simulink model "FDIA_Toolbox"  (R2018a)
settings: Solver=VariableStepAuto  StartTime=0.0  StopTime=10.0  RelTol=1e-3
libraries: commrandsrc3 x30, commutil2 x12, simulink_extras x6, simulink x4, commsynccomp2 x2, commanapbnd3 x2
(part 2 of 2)

== system FDIA_Toolbox/  /Attack Injected System2/valve ==
  control : Inport
  source flow : Inport  Port=2
  Limited Integrator : Subsystem  mask(Limited integrator.){lb=0, ub=1, xi=InitialPosition}
      mask prompts: lb "Lower bound:"; ub "Upper bound:"; xi "Initial condition"
      mask help: Limited integrator
      mask Help: Implements a limited integrator with \nan expression of the form:\n\nif(x<=lb and u<0) or (x>=ub and u>0)\n\txdot=0\nelse\n\txdot=u.
      mask Display: plot(-1,-0.2,3.5,1.2,[0.05,1,2,2.9],[0,0,1,1]);disp(' 1/s    ')
  Product : Product  SaturateOnIntegerOverflow=on  RndMeth=Zero  InputSameDT=on  OutDataTypeStr=Inherit: Same as first input
  out flow : Outport  InitialOutput=0
  wires:
  source flow/1 -> Product/2
  Product/1 -> out flow/1
  control/1 -> Limited Integrator/1(In_1)
  Limited Integrator/1(Out_1) -> Product/1

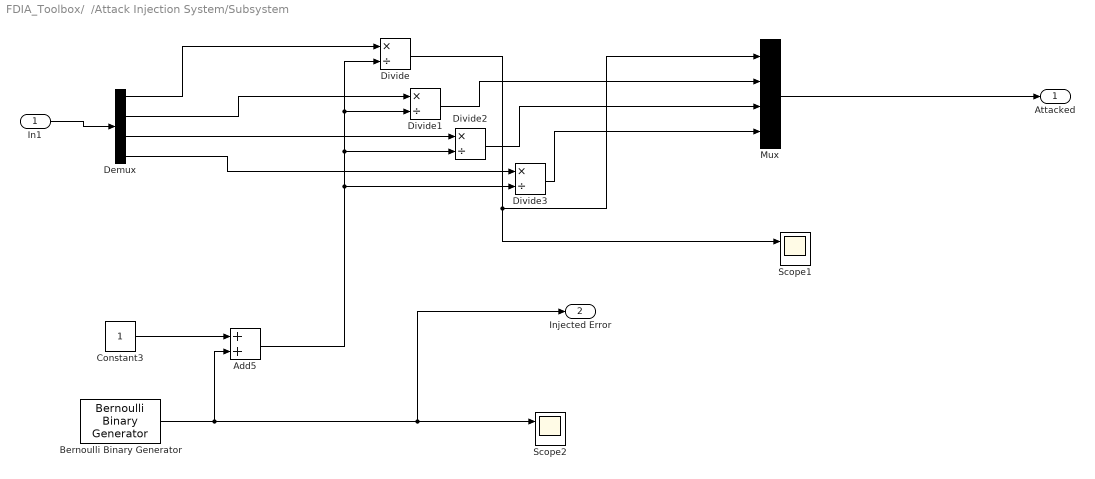
== system FDIA_Toolbox/  /Attack Injection System/Subsystem ==
  In1 : Inport
  Add5 : Sum  AccumDataTypeStr=uint8  RndMeth=Round
  Bernoulli Binary Generator : commrandsrc3/Bernoulli Binary Generator  ProbabilityOfZero=0.9  SeedSource=Auto  Seed=0  SampleTime=1  SamplesPerFrame=1  OutputDataType=uint8  SimulateUsing=Interpreted execution
  Constant3 : Constant  OutDataTypeStr=uint8
  Demux : Demux
  Divide{,1..3} (4 alike) : Product  Inputs=*/
  Mux : Mux
  Scope1 : Scope  NumInputPorts=2
  Scope2 : Scope  NumInputPorts=2
  Attacked : Outport
  Injected Error : Outport  Port=2
  wires:
  Demux/3 -> Divide2/1
  Demux/2 -> Divide1/1
  Demux/4 -> Divide3/1
  In1/1 -> Demux/1
  Mux/1 -> Attacked/1
  Divide/1 -> Scope1/1, Mux/1
  Bernoulli Binary Generator/1 -> Add5/2, Injected Error/1, Scope2/1
  Constant3/1 -> Add5/1
  Demux/1 -> Divide/1
  Add5/1 -> Divide3/2, Divide2/2, Divide1/2, Divide/2
  Divide1/1 -> Mux/2
  Divide2/1 -> Mux/3
  Divide3/1 -> Mux/4

== system FDIA_Toolbox/  /Attack Injection System1/tank  ==
  flow in : Inport
  1/area : Gain  Gain=1/area  SaturateOnIntegerOverflow=on  OutDataTypeStr=Inherit: Same as input  ParamDataTypeStr=Inherit: Same as input
  Overflow sensor1 : Relay  OnSwitchValue=ht - overflowLimit  OffSwitchValue=ht - overflowLimit  OnOutputValue=3  ZeroCross=off
  outletArea : Gain  Gain=outletArea  SaturateOnIntegerOverflow=on  OutDataTypeStr=Inherit: Same as input  ParamDataTypeStr=Inherit: Same as input
  sqrt(2gh) : Fcn  Expr=sqrt(2*9.8*u)
  sum : Sum  Inputs=+-  SaturateOnIntegerOverflow=on  InputSameDT=on  OutDataTypeStr=Inherit: Same as first input
  tank volume : Subsystem  mask(Limited integrator.){lb=0, ub=ht * area, xi=initialHt * area}
      mask prompts: lb "Lower bound:"; ub "Upper bound:"; xi "Initial condition"
      mask help: Limited integrator
      mask Help: Implements a limited integrator with \nan expression of the form:\n\nif(x<=lb and u<0) or (x>=ub and u>0)\n\txdot=0\nelse\n\txdot=u.
      mask Display: plot(-1,-0.2,3.5,1.2,[0.05,1,2,2.9],[0,0,1,1]);disp(' 1/s    ')
  water level : Outport  InitialOutput=0
  flow out : Outport  Port=2  InitialOutput=0
  overflow flag1 : Outport  Port=3  InitialOutput=0
  wires:
  outletArea/1 -> sum/2, flow out/1
  sqrt(2gh)/1 -> outletArea/1
  tank volume/1(Out_1) -> 1/area/1
  flow in/1 -> sum/1
  sum/1 -> tank volume/1(In_1)
  Overflow sensor1/1 -> overflow flag1/1
  1/area/1 -> sqrt(2gh)/1, Overflow sensor1/1, water level/1

== system FDIA_Toolbox/  /Attack Injection System1/valve ==
  control : Inport
  source flow : Inport  Port=2
  Limited Integrator : Subsystem  mask(Limited integrator.){lb=0, ub=1, xi=InitialPosition}
      mask prompts: lb "Lower bound:"; ub "Upper bound:"; xi "Initial condition"
      mask help: Limited integrator
      mask Help: Implements a limited integrator with \nan expression of the form:\n\nif(x<=lb and u<0) or (x>=ub and u>0)\n\txdot=0\nelse\n\txdot=u.
      mask Display: plot(-1,-0.2,3.5,1.2,[0.05,1,2,2.9],[0,0,1,1]);disp(' 1/s    ')
  Product : Product  SaturateOnIntegerOverflow=on  RndMeth=Zero  InputSameDT=on  OutDataTypeStr=Inherit: Same as first input
  out flow : Outport  InitialOutput=0
  wires:
  source flow/1 -> Product/2
  Product/1 -> out flow/1
  control/1 -> Limited Integrator/1(In_1)
  Limited Integrator/1(Out_1) -> Product/1

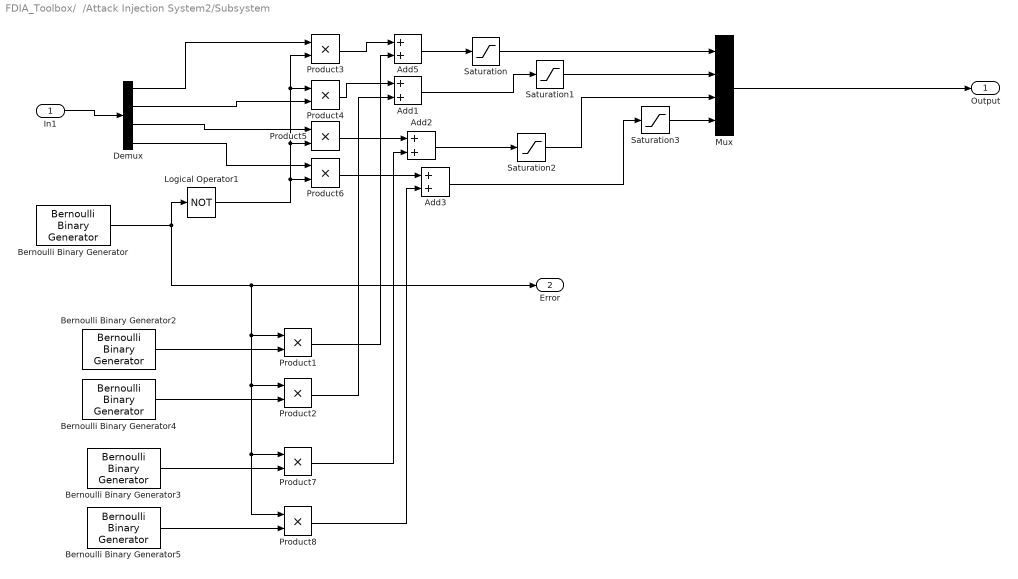
== system FDIA_Toolbox/  /Attack Injection System2/Subsystem ==
  In1 : Inport
  Add{1..3,5} (4 alike) : Sum  AccumDataTypeStr=uint8  RndMeth=Round
  Bernoulli Binary Generator : commrandsrc3/Bernoulli Binary Generator  ProbabilityOfZero=0.8  SeedSource=Auto  Seed=0  SampleTime=1  SamplesPerFrame=1  OutputDataType=uint8  SimulateUsing=Interpreted execution
  Bernoulli Binary Generator2 : commrandsrc3/Bernoulli Binary Generator  ProbabilityOfZero=0.1  SeedSource=Auto  Seed=0  SampleTime=1  SamplesPerFrame=1  OutputDataType=double  SimulateUsing=Interpreted execution
  Bernoulli Binary Generator3 : commrandsrc3/Bernoulli Binary Generator  ProbabilityOfZero=0.6  SeedSource=Auto  Seed=0  SampleTime=1  SamplesPerFrame=1  OutputDataType=double  SimulateUsing=Interpreted execution
  Bernoulli Binary Generator4 : commrandsrc3/Bernoulli Binary Generator  ProbabilityOfZero=0.4  SeedSource=Auto  Seed=0  SampleTime=1  SamplesPerFrame=1  OutputDataType=double  SimulateUsing=Interpreted execution
  Bernoulli Binary Generator5 : commrandsrc3/Bernoulli Binary Generator  ProbabilityOfZero=0.7  SeedSource=Auto  Seed=0  SampleTime=1  SamplesPerFrame=1  OutputDataType=double  SimulateUsing=Interpreted execution
  Demux : Demux
  Logical Operator1 : Logic  Operator=NOT  AllPortsSameDT=off  OutDataTypeStr=boolean
  Mux : Mux
  Product{1..8} (8 alike) : Product
  Saturation{,1..3} (4 alike) : Saturate  UpperLimit=1  LowerLimit=0
  Output : Outport
  Error : Outport  Port=2
  wires:
  Demux/3 -> Product5/1
  Demux/2 -> Product4/2
  Demux/4 -> Product6/1
  In1/1 -> Demux/1
  Mux/1 -> Output/1
  Bernoulli Binary Generator/1 -> Product8/1, Product7/1, Product2/1, Product1/1, Error/1, Logical Operator1/1
  Demux/1 -> Product3/1
  Logical Operator1/1 -> Product6/2, Product5/2, Product3/2, Product4/1
  Product3/1 -> Add5/1
  Product6/1 -> Add3/1
  Product5/1 -> Add2/1
  Product4/1 -> Add1/1
  Add5/1 -> Saturation/1
  Add1/1 -> Saturation1/1
  Add2/1 -> Saturation2/1
  Add3/1 -> Saturation3/1
  Saturation/1 -> Mux/1
  Saturation3/1 -> Mux/4
  Saturation2/1 -> Mux/3
  Saturation1/1 -> Mux/2
  Bernoulli Binary Generator5/1 -> Product8/2
  Product8/1 -> Add3/2
  Bernoulli Binary Generator3/1 -> Product7/2
  Product7/1 -> Add2/2
  Bernoulli Binary Generator4/1 -> Product2/2
  Product2/1 -> Add1/2
  Bernoulli Binary Generator2/1 -> Product1/2
  Product1/1 -> Add5/2

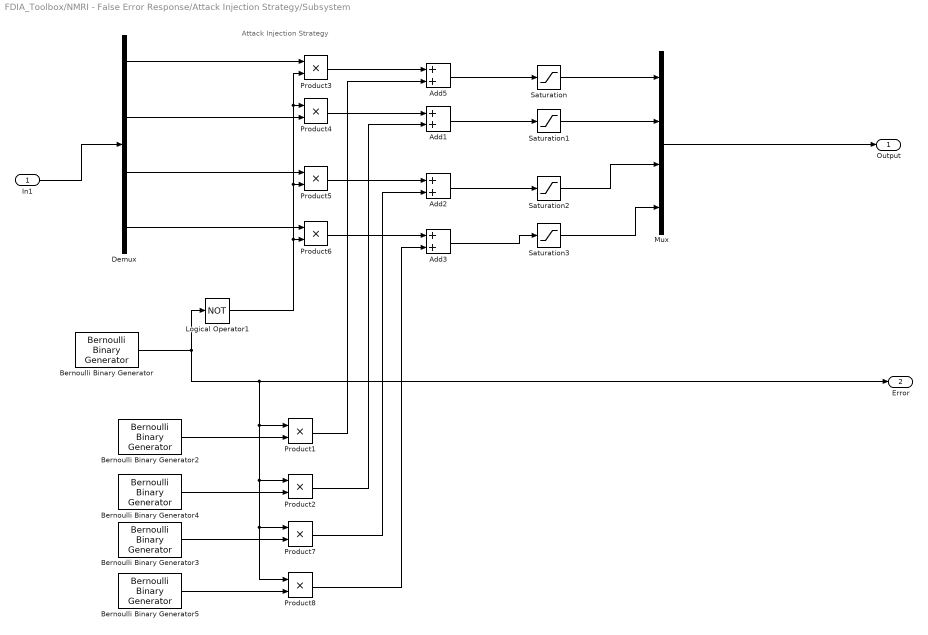
== system FDIA_Toolbox/NMRI - False Error Response/Attack Injection Strategy/Subsystem ==
  note: Attack Injection Strategy
  In1 : Inport
  Add{1..3,5} (4 alike) : Sum  AccumDataTypeStr=uint8  RndMeth=Round
  Bernoulli Binary Generator : commrandsrc3/Bernoulli Binary Generator  ProbabilityOfZero=0.8  SeedSource=Auto  Seed=0  SampleTime=1  SamplesPerFrame=1  OutputDataType=uint8  SimulateUsing=Interpreted execution
  Bernoulli Binary Generator2 : commrandsrc3/Bernoulli Binary Generator  ProbabilityOfZero=0.1  SeedSource=Auto  Seed=0  SampleTime=1  SamplesPerFrame=1  OutputDataType=double  SimulateUsing=Interpreted execution
  Bernoulli Binary Generator3 : commrandsrc3/Bernoulli Binary Generator  ProbabilityOfZero=0.6  SeedSource=Auto  Seed=0  SampleTime=1  SamplesPerFrame=1  OutputDataType=double  SimulateUsing=Interpreted execution
  Bernoulli Binary Generator4 : commrandsrc3/Bernoulli Binary Generator  ProbabilityOfZero=0.4  SeedSource=Auto  Seed=0  SampleTime=1  SamplesPerFrame=1  OutputDataType=double  SimulateUsing=Interpreted execution
  Bernoulli Binary Generator5 : commrandsrc3/Bernoulli Binary Generator  ProbabilityOfZero=0.7  SeedSource=Auto  Seed=0  SampleTime=1  SamplesPerFrame=1  OutputDataType=double  SimulateUsing=Interpreted execution
  Demux : Demux
  Logical Operator1 : Logic  Operator=NOT  AllPortsSameDT=off  OutDataTypeStr=boolean
  Mux : Mux
  Product{1..8} (8 alike) : Product
  Saturation{,1..3} (4 alike) : Saturate  UpperLimit=1  LowerLimit=0
  Output : Outport
  Error : Outport  Port=2
  wires:
  Demux/3 -> Product5/1
  Demux/2 -> Product4/2
  Demux/4 -> Product6/1
  In1/1 -> Demux/1
  Mux/1 -> Output/1
  Bernoulli Binary Generator/1 -> Logical Operator1/1, Product8/1, Product7/1, Product2/1, Product1/1, Error/1
  Demux/1 -> Product3/1
  Logical Operator1/1 -> Product6/2, Product5/2, Product3/2, Product4/1
  Product3/1 -> Add5/1
  Product6/1 -> Add3/1
  Product5/1 -> Add2/1
  Product4/1 -> Add1/1
  Add5/1 -> Saturation/1
  Add1/1 -> Saturation1/1
  Add2/1 -> Saturation2/1
  Add3/1 -> Saturation3/1
  Saturation/1 -> Mux/1
  Saturation3/1 -> Mux/4
  Saturation2/1 -> Mux/3
  Saturation1/1 -> Mux/2
  Bernoulli Binary Generator5/1 -> Product8/2
  Product8/1 -> Add3/2
  Bernoulli Binary Generator3/1 -> Product7/2
  Product7/1 -> Add2/2
  Bernoulli Binary Generator4/1 -> Product2/2
  Product2/1 -> Add1/2
  Bernoulli Binary Generator2/1 -> Product1/2
  Product1/1 -> Add5/2

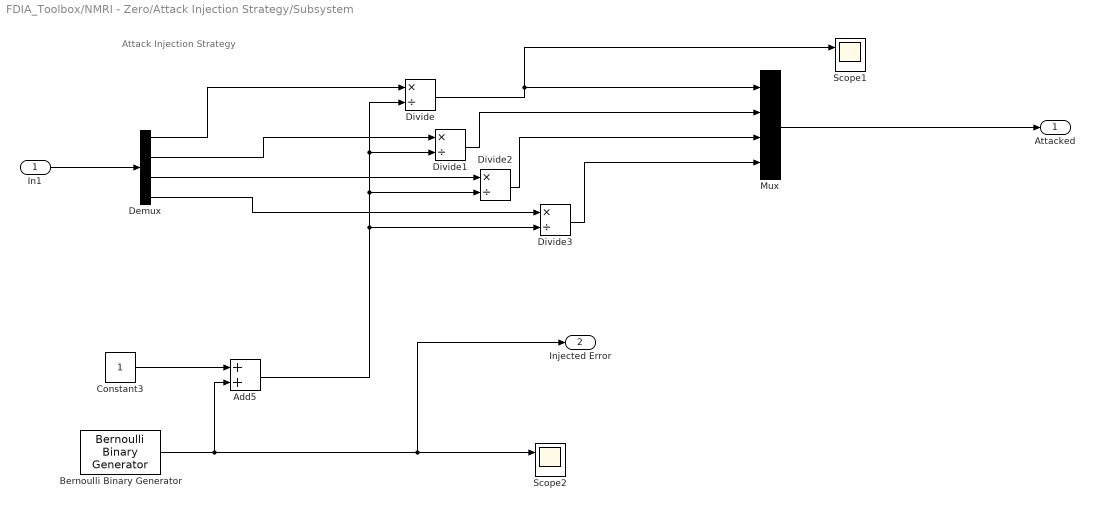
== system FDIA_Toolbox/NMRI - Zero/Attack Injection Strategy/Subsystem ==
  note: Attack Injection Strategy
  In1 : Inport
  Add5 : Sum  AccumDataTypeStr=uint8  RndMeth=Round
  Bernoulli Binary Generator : commrandsrc3/Bernoulli Binary Generator  ProbabilityOfZero=0.9  SeedSource=Auto  Seed=0  SampleTime=1  SamplesPerFrame=1  OutputDataType=uint8  SimulateUsing=Interpreted execution
  Constant3 : Constant  OutDataTypeStr=uint8
  Demux : Demux
  Divide{,1..3} (4 alike) : Product  Inputs=*/
  Mux : Mux
  Scope1 : Scope  NumInputPorts=2
  Scope2 : Scope  NumInputPorts=2
  Attacked : Outport
  Injected Error : Outport  Port=2
  wires:
  Demux/3 -> Divide2/1
  Demux/2 -> Divide1/1
  Demux/4 -> Divide3/1
  In1/1 -> Demux/1
  Mux/1 -> Attacked/1
  Divide/1 -> Mux/1, Scope1/1
  Bernoulli Binary Generator/1 -> Add5/2, Injected Error/1, Scope2/1
  Constant3/1 -> Add5/1
  Demux/1 -> Divide/1
  Add5/1 -> Divide3/2, Divide2/2, Divide1/2, Divide/2
  Divide1/1 -> Mux/2
  Divide2/1 -> Mux/3
  Divide3/1 -> Mux/4

== system FDIA_Toolbox/NMRI- Ones/Attack Induced Strategy/Subsystem ==
  note: Attack Injection Strategy
  In1 : Inport
  Demux : Demux
  Mux : Mux
  Saturation{,1..3} (4 alike) : Saturate  UpperLimit=1  LowerLimit=0
  Attacked Injection : Outport
  wires:
  Demux/3 -> Saturation2/1
  Demux/2 -> Saturation1/1
  In1/1 -> Demux/1
  Mux/1 -> Attacked Injection/1
  Demux/1 -> Saturation/1
  Demux/4 -> Saturation3/1
  Saturation/1 -> Mux/1
  Saturation3/1 -> Mux/4
  Saturation2/1 -> Mux/3
  Saturation1/1 -> Mux/2

== system FDIA_Toolbox/  /Attack Induced System1/tank /tank volume ==
  In_1 : Inport
  Fcn : Fcn  Expr=u[2]*((((u[1]>lb)+(u[2]>=0))>0) * (((u[1]<ub)+(u[2]<=0))>0))
  Integrator : Integrator  InitialCondition=xi
  Mux : Mux  Inputs=2
  Saturation : Saturate  UpperLimit=ub  LowerLimit=lb  ZeroCross=off
  Out_1 : Outport  InitialOutput=0
  wires:
  Integrator/1 -> Saturation/1, Mux/1
  Fcn/1 -> Integrator/1
  Mux/1 -> Fcn/1
  In_1/1 -> Mux/2
  Saturation/1 -> Out_1/1

== system FDIA_Toolbox/  /Attack Induced System1/valve/Limited Integrator ==
  In_1 : Inport
  Fcn : Fcn  Expr=u[2]*((((u[1]>lb)+(u[2]>=0))>0) * (((u[1]<ub)+(u[2]<=0))>0))
  Integrator : Integrator  InitialCondition=xi
  Mux : Mux  Inputs=2
  Saturation : Saturate  UpperLimit=ub  LowerLimit=lb  ZeroCross=off
  Out_1 : Outport  InitialOutput=0
  wires:
  Integrator/1 -> Saturation/1, Mux/1
  Fcn/1 -> Integrator/1
  Mux/1 -> Fcn/1
  In_1/1 -> Mux/2
  Saturation/1 -> Out_1/1

== system FDIA_Toolbox/  /Attack Injected System/tank /tank volume ==
  In_1 : Inport
  Fcn : Fcn  Expr=u[2]*((((u[1]>lb)+(u[2]>=0))>0) * (((u[1]<ub)+(u[2]<=0))>0))
  Integrator : Integrator  InitialCondition=xi
  Mux : Mux  Inputs=2
  Saturation : Saturate  UpperLimit=ub  LowerLimit=lb  ZeroCross=off
  Out_1 : Outport  InitialOutput=0
  wires:
  Integrator/1 -> Saturation/1, Mux/1
  Fcn/1 -> Integrator/1
  Mux/1 -> Fcn/1
  In_1/1 -> Mux/2
  Saturation/1 -> Out_1/1

== system FDIA_Toolbox/  /Attack Injected System/valve/Limited Integrator ==
  In_1 : Inport
  Fcn : Fcn  Expr=u[2]*((((u[1]>lb)+(u[2]>=0))>0) * (((u[1]<ub)+(u[2]<=0))>0))
  Integrator : Integrator  InitialCondition=xi
  Mux : Mux  Inputs=2
  Saturation : Saturate  UpperLimit=ub  LowerLimit=lb  ZeroCross=off
  Out_1 : Outport  InitialOutput=0
  wires:
  Integrator/1 -> Saturation/1, Mux/1
  Fcn/1 -> Integrator/1
  Mux/1 -> Fcn/1
  In_1/1 -> Mux/2
  Saturation/1 -> Out_1/1

== system FDIA_Toolbox/  /Attack Injected System2/Original System/tank 1 ==
  flow in : Inport
  1/area : Gain  Gain=1/area  SaturateOnIntegerOverflow=on  OutDataTypeStr=Inherit: Same as input  ParamDataTypeStr=Inherit: Same as input
  Overflow sensor1 : Relay  OnSwitchValue=ht - overflowLimit  OffSwitchValue=ht - overflowLimit  OnOutputValue=3  ZeroCross=off
  outletArea : Gain  Gain=outletArea  SaturateOnIntegerOverflow=on  OutDataTypeStr=Inherit: Same as input  ParamDataTypeStr=Inherit: Same as input
  sqrt(2gh) : Fcn  Expr=sqrt(2*9.8*u)
  sum : Sum  Inputs=+-  SaturateOnIntegerOverflow=on  InputSameDT=on  OutDataTypeStr=Inherit: Same as first input
  tank volume : Subsystem  mask(Limited integrator.){lb=0, ub=ht * area, xi=initialHt * area}
      mask prompts: lb "Lower bound:"; ub "Upper bound:"; xi "Initial condition"
      mask help: Limited integrator
      mask Help: Implements a limited integrator with \nan expression of the form:\n\nif(x<=lb and u<0) or (x>=ub and u>0)\n\txdot=0\nelse\n\txdot=u.
      mask Display: plot(-1,-0.2,3.5,1.2,[0.05,1,2,2.9],[0,0,1,1]);disp(' 1/s    ')
  water level : Outport  InitialOutput=0
  flow out : Outport  Port=2  InitialOutput=0
  overflow flag1 : Outport  Port=3  InitialOutput=0
  wires:
  outletArea/1 -> sum/2, flow out/1
  sqrt(2gh)/1 -> outletArea/1
  tank volume/1(Out_1) -> 1/area/1
  flow in/1 -> sum/1
  sum/1 -> tank volume/1(In_1)
  Overflow sensor1/1 -> overflow flag1/1
  1/area/1 -> sqrt(2gh)/1, Overflow sensor1/1, water level/1

== system FDIA_Toolbox/  /Attack Injected System2/Original System/valve1 ==
  control : Inport
  source flow : Inport  Port=2
  Limited Integrator : Subsystem  mask(Limited integrator.){lb=0, ub=1, xi=InitialPosition}
      mask prompts: lb "Lower bound:"; ub "Upper bound:"; xi "Initial condition"
      mask help: Limited integrator
      mask Help: Implements a limited integrator with \nan expression of the form:\n\nif(x<=lb and u<0) or (x>=ub and u>0)\n\txdot=0\nelse\n\txdot=u.
      mask Display: plot(-1,-0.2,3.5,1.2,[0.05,1,2,2.9],[0,0,1,1]);disp(' 1/s    ')
  Product : Product  SaturateOnIntegerOverflow=on  RndMeth=Zero  InputSameDT=on  OutDataTypeStr=Inherit: Same as first input
  out flow : Outport  InitialOutput=0
  wires:
  source flow/1 -> Product/2
  Product/1 -> out flow/1
  control/1 -> Limited Integrator/1(In_1)
  Limited Integrator/1(Out_1) -> Product/1

== system FDIA_Toolbox/  /Attack Injected System2/tank /tank volume ==
  In_1 : Inport
  Fcn : Fcn  Expr=u[2]*((((u[1]>lb)+(u[2]>=0))>0) * (((u[1]<ub)+(u[2]<=0))>0))
  Integrator : Integrator  InitialCondition=xi
  Mux : Mux  Inputs=2
  Saturation : Saturate  UpperLimit=ub  LowerLimit=lb  ZeroCross=off
  Out_1 : Outport  InitialOutput=0
  wires:
  Integrator/1 -> Saturation/1, Mux/1
  Fcn/1 -> Integrator/1
  Mux/1 -> Fcn/1
  In_1/1 -> Mux/2
  Saturation/1 -> Out_1/1

== system FDIA_Toolbox/  /Attack Injected System2/valve/Limited Integrator ==
  In_1 : Inport
  Fcn : Fcn  Expr=u[2]*((((u[1]>lb)+(u[2]>=0))>0) * (((u[1]<ub)+(u[2]<=0))>0))
  Integrator : Integrator  InitialCondition=xi
  Mux : Mux  Inputs=2
  Saturation : Saturate  UpperLimit=ub  LowerLimit=lb  ZeroCross=off
  Out_1 : Outport  InitialOutput=0
  wires:
  Integrator/1 -> Saturation/1, Mux/1
  Fcn/1 -> Integrator/1
  Mux/1 -> Fcn/1
  In_1/1 -> Mux/2
  Saturation/1 -> Out_1/1

== system FDIA_Toolbox/  /Attack Injection System1/tank /tank volume ==
  In_1 : Inport
  Fcn : Fcn  Expr=u[2]*((((u[1]>lb)+(u[2]>=0))>0) * (((u[1]<ub)+(u[2]<=0))>0))
  Integrator : Integrator  InitialCondition=xi
  Mux : Mux  Inputs=2
  Saturation : Saturate  UpperLimit=ub  LowerLimit=lb  ZeroCross=off
  Out_1 : Outport  InitialOutput=0
  wires:
  Integrator/1 -> Saturation/1, Mux/1
  Fcn/1 -> Integrator/1
  Mux/1 -> Fcn/1
  In_1/1 -> Mux/2
  Saturation/1 -> Out_1/1

== system FDIA_Toolbox/  /Attack Injection System1/valve/Limited Integrator ==
  In_1 : Inport
  Fcn : Fcn  Expr=u[2]*((((u[1]>lb)+(u[2]>=0))>0) * (((u[1]<ub)+(u[2]<=0))>0))
  Integrator : Integrator  InitialCondition=xi
  Mux : Mux  Inputs=2
  Saturation : Saturate  UpperLimit=ub  LowerLimit=lb  ZeroCross=off
  Out_1 : Outport  InitialOutput=0
  wires:
  Integrator/1 -> Saturation/1, Mux/1
  Fcn/1 -> Integrator/1
  Mux/1 -> Fcn/1
  In_1/1 -> Mux/2
  Saturation/1 -> Out_1/1

== system FDIA_Toolbox/  /Attack Injected System2/Original System/tank 1/tank volume ==
  In_1 : Inport
  Fcn : Fcn  Expr=u[2]*((((u[1]>lb)+(u[2]>=0))>0) * (((u[1]<ub)+(u[2]<=0))>0))
  Integrator : Integrator  InitialCondition=xi
  Mux : Mux  Inputs=2
  Saturation : Saturate  UpperLimit=ub  LowerLimit=lb  ZeroCross=off
  Out_1 : Outport  InitialOutput=0
  wires:
  Integrator/1 -> Saturation/1, Mux/1
  Fcn/1 -> Integrator/1
  Mux/1 -> Fcn/1
  In_1/1 -> Mux/2
  Saturation/1 -> Out_1/1

== system FDIA_Toolbox/  /Attack Injected System2/Original System/valve1/Limited Integrator ==
  In_1 : Inport
  Fcn : Fcn  Expr=u[2]*((((u[1]>lb)+(u[2]>=0))>0) * (((u[1]<ub)+(u[2]<=0))>0))
  Integrator : Integrator  InitialCondition=xi
  Mux : Mux  Inputs=2
  Saturation : Saturate  UpperLimit=ub  LowerLimit=lb  ZeroCross=off
  Out_1 : Outport  InitialOutput=0
  wires:
  Integrator/1 -> Saturation/1, Mux/1
  Fcn/1 -> Integrator/1
  Mux/1 -> Fcn/1
  In_1/1 -> Mux/2
  Saturation/1 -> Out_1/1

== matlab function FDIA_Toolbox/MFCI - Force Lister Only Mode /MATLAB Function ==
  data: varargin input; varargout output
function varargout = fcn(varargin)
unction varargout = Final_14MFCI(varargin)
% FINAL_14MFCI MATLAB code for Final_14MFCI.fig
%      FINAL_14MFCI, by itself, creates a new FINAL_14MFCI or raises the existing
%      singleton*.
%
%      H = FINAL_14MFCI returns the handle to a new FINAL_14MFCI or the handle to
%      the existing singleton*.
%
%      FINAL_14MFCI('CALLBACK',hObject,eventData,handles,...) calls the local
%      function named CALLBACK in FINAL_14MFCI.M with the given input arguments.
%
%      FINAL_14MFCI('Property','Value',...) creates a new FINAL_14MFCI or raises the
%      existing singleton*.  Starting from the left, property value pairs are
%      applied to the GUI before Final_14MFCI_OpeningFcn gets called.  An
%      unrecognized property name or invalid value makes property application
%      stop.  All inputs are passed to Final_14MFCI_OpeningFcn via varargin.
%
%      *See GUI Options on GUIDE's Tools menu.  Choose "GUI allows only one
%      instance to run (singleton)".
%
% See also: GUIDE, GUIDATA, GUIHANDLES

% Edit the above text to modify the response to help Final_14MFCI

% Last Modified by GUIDE v2.5 06-Mar-2018 15:16:01

% Begin initialization code - DO NOT EDIT
gui_Singleton = 1;
gui_State = struct('gui_Name',       mfilename, ...
                   'gui_Singleton',  gui_Singleton, ...
                   'gui_OpeningFcn', @Final_14MFCI_OpeningFcn, ...
                   'gui_OutputFcn',  @Final_14MFCI_OutputFcn, ...
                   'gui_LayoutFcn',  [] , ...
                   'gui_Callback',   []);
if nargin && ischar(varargin{1})
    gui_State.gui_Callback = str2func(varargin{1});
end

if nargout
    [varargout{1:nargout}] = gui_mainfcn(gui_State, varargin{:});
else
    gui_mainfcn(gui_State, varargin{:});
end
% End initialization code - DO NOT EDIT


% --- Executes just before Final_14MFCI is made visible.
function Final_14MFCI_OpeningFcn(hObject, eventdata, handles, varargin)
% This function has no output args, see OutputFcn.
% hObject    handle to figure
% eventdata  reserved - to be defined in a future version of MATLAB
% handles    structure with handles and user data (see GUIDATA)
% varargin   command line arguments to Final_14MFCI (see VARARGIN)

% Choose default command line output for Final_14MFCI
handles.output = hObject;

% Update handles structure
guidata(hObject, handles);

% UIWAIT makes Final_14MFCI wait for user response (see UIRESUME)
% uiwait(handles.figure1);


% --- Outputs from this function are returned to the command line.
function varargout = Final_14MFCI_OutputFcn(hObject, eventdata, handles) 
% varargout  cell array for returning output args (see VARARGOUT);
% hObject    handle to figure
% eventdata  reserved - to be defined in a future version of MATLAB
% handles    structure with handles and user data (see GUIDATA)

% Get default command line output from handles structure
varargout{1} = handles.output;
global x;
x = 0:0.1:100;
global counter;
counter = 0;


% --- Executes on button press in sine.
function sine_Callback(hObject, eventdata, handles)
% hObject    handle to sine (see GCBO)
% eventdata  reserved - to be defined in a future version of MATLAB
% handles    structure with handles and user data (see GUIDATA)
xlabel ('Time');                                                    %labels the x axis
ylabel ('Frequency');                                               %labels the y axis
title ('Sine Signal');
global x;
global counter;
f=sin(x);
curve = animatedline;
set(gca,'XLim',[0 100],'YLim',[-1 1]);
set(handles.stop, 'userdata', 0);
for i = 1:length(x)
    counter = counter + 1;
    addpoints(curve, x(i), f(i));
    drawnow;
    if get(handles.stop, 'userdata') % stop condition
         break; 
    end
end
   
% --- Executes on button press in attack.
function attack_Callback(hObject, eventdata, handles)
% hObject    handle to attack (see GCBO)
% eventdata  reserved - to be defined in a future version of MATLAB
% handles    structure with handles and user data (see GUIDATA)

xlabel ('Time');                                                    %labels the x axis
ylabel ('Frequency');                                               %labels the y axis
title ('Attacked Signal');
global x;
global counter;
yn = rand(size(x));                       
curve = animatedline;
set(gca,'XLim',[0 100],'YLim',[-1 1]);
for j= counter:length(x)
    addpoints(curve,x(j),yn(j));
    drawnow
end

% --- Executes on button press in stop.
function stop_Callback(hObject, eventdata, handles)
% hObject    handle to stop (see GCBO)
% eventdata  reserved - to be defined in a future version of MATLAB
% handles    structure with handles and user data (see GUIDATA)
set(handles.stop, 'userdata', 1);
